simulink model "controller_arduino_4_mahdy_f"  (R2024a)
settings: Solver=FixedStepDiscrete  StartTime=0.0  StopTime=inf  FixedStep=0.01  RelTol=1e-3  EnableMultiTasking=on
libraries: arduinolib x15
settings Model: ExtModeTrigDuration=2  Creator=mahdy  LastModifiedBy=mahdy
settings SolverCC: AutoInsertRateTranBlk=on
settings OptimizationCC: EnhancedBackFolding=on  PassReuseOutputArgsAs=Individual arguments  ZeroExternalMemoryAtStartup=off  ZeroInternalMemoryAtStartup=off  MaxStackSize=64  OptimizeBlockOrder=speed  DifferentSizesBufferReuse=on  OptimizationCustomize=off  EfficientTunableParamExpr=on
settings DebuggingCC: ParameterTunabilityLossMsg=error
settings HardwareCC: ProdBitPerInt=16  ProdBitPerPointer=16  ProdBitPerSizeT=16  ProdBitPerPtrDiffT=16  ProdLargestAtomicFloat=None  ProdWordSize=8  ProdHWDeviceType=Atmel->AVR
settings SFSimCC: MATLABDynamicMemAlloc=off
settings RTWCC: Description=Embedded Coder  SystemTargetFile=ert.tlc  HardwareBoard=Arduino Uno  TemplateMakefile=ert_default_tmf  Toolchain=Arduino AVR  BuildConfiguration=Faster Runs
settings CodeAppCC: ForceParamTrailComments=on  IgnoreCustomStorageClasses=off  OperatorAnnotations=on  SimulinkDataObjDesc=on  SFDataObjDesc=on  InsertBlockDesc=on
settings ERTTargetCC: SupportContinuousTime=on  SupportVariableSizeSignals=on  ExtModeTransport=3  ExtModeStaticAlloc=on  ExtModeAutomaticAllocSize=off  ExtModeStaticAllocSize=250  ExtModeMexFile=ext_xcp  ExtModeIntrfLevel=Level2 - Open

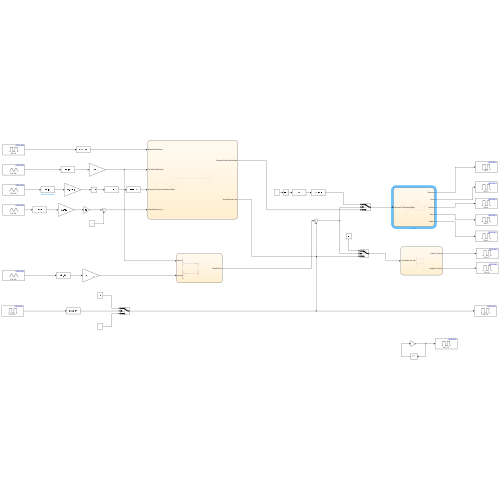
[thumbnail: Simulink's stored preview of the top-level diagram]
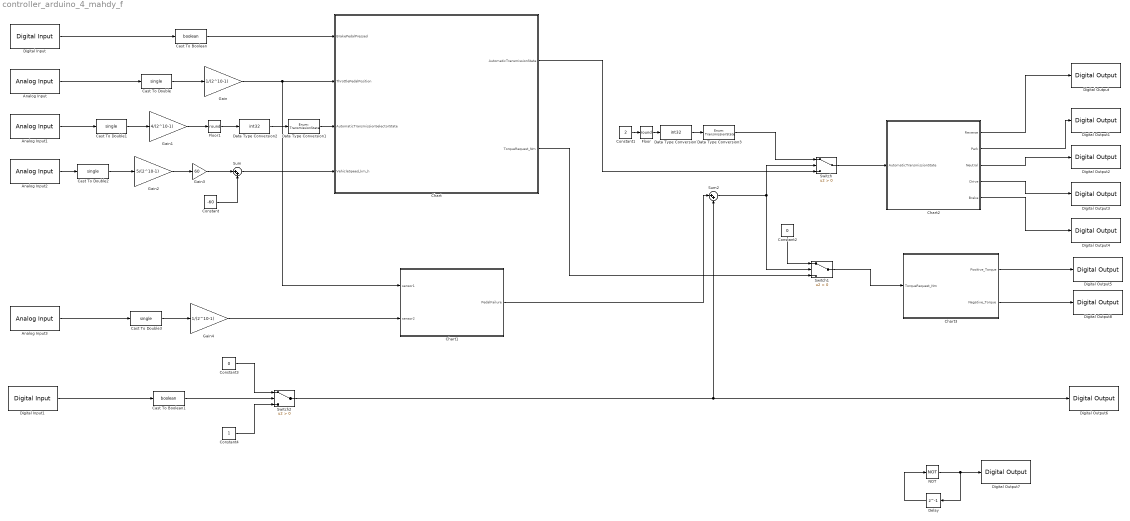
== system controller_arduino_4_mahdy_f ==
  Analog Input : arduinolib/Analog Input  pinNumber=2  ReadResultsOnly=off  ConversionTriggerSource=Software  ExternalTriggerType=uint32( 0 )  OutputDataType=uint16  EnableConversionCompleteNotify=off  EnableOuputStatus=off  SampleTime=-1  blockPlatform=arduino
  Analog Input1 : arduinolib/Analog Input  pinNumber=3  ReadResultsOnly=off  ConversionTriggerSource=Software  ExternalTriggerType=uint32( 0 )  OutputDataType=uint16  EnableConversionCompleteNotify=off  EnableOuputStatus=off  SampleTime=-1  blockPlatform=arduino
  Analog Input2 : arduinolib/Analog Input  pinNumber=4  ReadResultsOnly=off  ConversionTriggerSource=Software  ExternalTriggerType=uint32( 0 )  OutputDataType=uint16  EnableConversionCompleteNotify=off  EnableOuputStatus=off  SampleTime=-1  blockPlatform=arduino
  Analog Input3 : arduinolib/Analog Input  pinNumber=5  ReadResultsOnly=off  ConversionTriggerSource=Software  ExternalTriggerType=uint32( 0 )  OutputDataType=uint16  EnableConversionCompleteNotify=off  EnableOuputStatus=off  SampleTime=-1  blockPlatform=arduino
  Cast To Boolean : DataTypeConversion  OutDataTypeStr=boolean  SaturateOnIntegerOverflow=off  RndMeth=Floor
  Cast To Boolean1 : DataTypeConversion  OutDataTypeStr=boolean  SaturateOnIntegerOverflow=off  RndMeth=Floor
  Cast To Double{,1..3} (4 alike) : DataTypeConversion  OutDataTypeStr=single  SaturateOnIntegerOverflow=off  RndMeth=Floor
  Chart : Stateflow chart  TreatAsAtomicUnit=on
  Chart1 : Stateflow chart  TreatAsAtomicUnit=on
  Chart2 : Stateflow chart  TreatAsAtomicUnit=on
  Chart3 : Stateflow chart  TreatAsAtomicUnit=on
  Constant : Constant  Value=-60  OutDataTypeStr=single
  Constant1 : Constant  Value=2
  Constant2 : Constant  Value=0
  Constant3 : Constant  Value=0
  Constant4 : Constant
  Data Type Conversion1 : DataTypeConversion  OutDataTypeStr=Enum: TransmissionState  SaturateOnIntegerOverflow=off  RndMeth=Floor  LockScale=on
  Data Type Conversion2 : DataTypeConversion  OutDataTypeStr=int32  SaturateOnIntegerOverflow=off  RndMeth=Floor  LockScale=on
  Data Type Conversion3 : DataTypeConversion  OutDataTypeStr=Enum: TransmissionState  SaturateOnIntegerOverflow=off  RndMeth=Floor  LockScale=on
  Data Type Conversion7 : DataTypeConversion  OutDataTypeStr=int32  SaturateOnIntegerOverflow=off  RndMeth=Floor  LockScale=on
  Delay : Delay  DelayLength=1  SampleTime=0.01
  Digital Input : arduinolib/Digital Input  pinNumber=8  mode=Default  Direction=input  SampleTime=0.1  blockPlatform=arduino
  Digital Input1 : arduinolib/Digital Input  pinNumber=10  mode=Default  Direction=input  SampleTime=0.1  blockPlatform=arduino
  Digital Output : arduinolib/Digital Output  pinNumber=2  Direction=output  blockPlatform=arduino
  Digital Output1 : arduinolib/Digital Output  pinNumber=3  Direction=output  blockPlatform=arduino
  Digital Output2 : arduinolib/Digital Output  pinNumber=4  Direction=output  blockPlatform=arduino
  Digital Output3 : arduinolib/Digital Output  pinNumber=5  Direction=output  blockPlatform=arduino
  Digital Output4 : arduinolib/Digital Output  pinNumber=6  Direction=output  blockPlatform=arduino
  Digital Output5 : arduinolib/Digital Output  pinNumber=7  Direction=output  blockPlatform=arduino
  Digital Output6 : arduinolib/Digital Output  pinNumber=12  Direction=output  blockPlatform=arduino
  Digital Output7 : arduinolib/Digital Output  pinNumber=13  Direction=output  blockPlatform=arduino
  Digital Output8 : arduinolib/Digital Output  pinNumber=9  Direction=output  blockPlatform=arduino
  Floor : Rounding  Operator=round
  Floor1 : Rounding  Operator=round
  Gain : Gain  Gain=1/(2^10-1)
  Gain1 : Gain  Gain=4/(2^10-1)
  Gain2 : Gain  Gain=5/(2^10-1)
  Gain3 : Gain  Gain=60
  Gain4 : Gain  Gain=1/(2^10-1)
  NOT : Logic  Operator=NOT  IconShape=distinctive  AllPortsSameDT=off  OutDataTypeStr=boolean
  Sum : Sum  Inputs=|++
  Sum2 : Sum  Inputs=|++
  Switch : Switch  Criteria=u2 > Threshold  SaturateOnIntegerOverflow=off  InputSameDT=off
  Switch1 : Switch  Criteria=u2 > Threshold  SaturateOnIntegerOverflow=off  InputSameDT=off
  Switch2 : Switch  Criteria=u2 > Threshold  SaturateOnIntegerOverflow=off  InputSameDT=off
  wires:
  Digital Input/1 -> Cast To Boolean/1
  Cast To Boolean/1 -> Chart/1(BrakePedalPressed)
  Analog Input/1 -> Cast To Double/1
  Cast To Double/1 -> Gain/1
  Analog Input1/1 -> Cast To Double1/1
  Gain/1 -> Chart1/1(sensor1), Chart/2(ThrottlePedalPosition)
  Cast To Double1/1 -> Gain1/1
  Data Type Conversion2/1 -> Data Type Conversion1/1
  Floor1/1 -> Data Type Conversion2/1
  Data Type Conversion1/1 -> Chart/3(AutomaticTransmissionSelectorState)
  Gain1/1 -> Floor1/1
  Analog Input2/1 -> Cast To Double2/1
  Gain2/1 -> Gain3/1
  Cast To Double2/1 -> Gain2/1
  Gain3/1 -> Sum/1
  Constant/1 -> Sum/2
  Sum/1 -> Chart/4(VehicleSpeed_km_h)
  Analog Input3/1 -> Cast To Double3/1
  Cast To Double3/1 -> Gain4/1
  Gain4/1 -> Chart1/2(sensor2)
  Constant2/1 -> Switch1/1
  Data Type Conversion3/1 -> Switch/1
  Sum2/1 -> Switch/2, Switch1/2
  Data Type Conversion7/1 -> Data Type Conversion3/1
  Chart1/1(PedalFailure) -> Sum2/1
  Chart/2(TorqueRequest_Nm) -> Switch1/3
  Chart/1(AutomaticTransmissionState) -> Switch/3
  NOT/1 -> Delay/1, Digital Output7/1
  Delay/1 -> NOT/1
  Digital Input1/1 -> Cast To Boolean1/1
  Constant3/1 -> Switch2/1
  Constant4/1 -> Switch2/3
  Switch2/1 -> Digital Output6/1, Sum2/2
  Chart3/2(Negative_Torque) -> Digital Output8/1
  Chart3/1(Positive_Torque) -> Digital Output5/1
  Switch1/1 -> Chart3/1(TorqueRequest_Nm)
  Switch/1 -> Chart2/1(AutomaticTransmissionState)
  Chart2/2(Park) -> Digital Output1/1
  Chart2/3(Neutral) -> Digital Output2/1
  Chart2/1(Reverse) -> Digital Output/1
  Chart2/5(Brake) -> Digital Output4/1
  Constant1/1 -> Floor/1
  Floor/1 -> Data Type Conversion7/1
  Chart2/4(Drive) -> Digital Output3/1
  Cast To Boolean1/1 -> Switch2/2

== stateflow chart controller_arduino_4_mahdy_f/Chart2 ==
  settings: updateMethod=DISCRETE  sampleTime=0.1
  state ReverseState
    entry:
    Reverse = 1
  state BrakeState
    entry:
    Brake = 1
  state ParkState
    entry:
    Park = 1
  state Input_transmissionState
  state NeutralState
    entry:
    Neutral = 1
  state DriveState
    entry:
    Drive = 1
  ReverseState -> Input_transmissionState : [AutomaticTransmissionState ~= TransmissionState.Reverse]{Reverse = 0}
  Input_transmissionState -> ReverseState [order 1] : [AutomaticTransmissionState == TransmissionState.Reverse]
  (default) -> Input_transmissionState
  Input_transmissionState -> BrakeState [order 5] : [AutomaticTransmissionState == TransmissionState.Brake]
  BrakeState -> Input_transmissionState : [AutomaticTransmissionState ~= TransmissionState.Brake]{Brake = 0}
  Input_transmissionState -> ParkState [order 2] : [AutomaticTransmissionState == TransmissionState.Park]
  ParkState -> Input_transmissionState : [AutomaticTransmissionState ~= TransmissionState.Park]{Park = 0}
  Input_transmissionState -> DriveState [order 4] : [AutomaticTransmissionState == TransmissionState.Drive]
  DriveState -> Input_transmissionState : [AutomaticTransmissionState ~= TransmissionState.Drive]{Drive = 0}
  Input_transmissionState -> NeutralState [order 3] : [AutomaticTransmissionState == TransmissionState.Neutral]
  NeutralState -> Input_transmissionState : [AutomaticTransmissionState ~= TransmissionState.Neutral]{Neutral = 0}
  data: AutomaticTransmissionState input; Reverse output =0; Park output =0; Neutral output =0; Drive output =0; Brake output =0

== stateflow chart controller_arduino_4_mahdy_f/Chart ==
  settings: updateMethod=DISCRETE  sampleTime=0.1
  state Reverse
    entry:
    AutomaticTransmissionState =TransmissionState. Reverse;
    during:
    TorqueRequest_Nm = -ThrottlePedalPosition*MAX_TORQUE_REVERSE;
  state Park
    entry:
    AutomaticTransmissionState = TransmissionState.Park;
    TorqueRequest_Nm = 0;
  state Neutral
    entry:
    AutomaticTransmissionState = TransmissionState.Neutral;
    TorqueRequest_Nm = 0;
  state Bmode
    entry:
    AutomaticTransmissionState = TransmissionState.Brake;
    state Acceleration
      during:
      TorqueRequest_Nm =MAX_TORQUE*(ThrottlePedalPosition-1/3)*3/2;
    state Regenerative_Braking
      during:
      TorqueRequest_Nm =- MAX_TORQUE*(1-3*ThrottlePedalPosition)
    state Stop
      entry:
      TorqueRequest_Nm = 0;
    (default) -> Acceleration
    Acceleration -> Regenerative_Braking : [ThrottlePedalPosition<=1/3]
    Regenerative_Braking -> Acceleration [order 1] : [ThrottlePedalPosition>1/3]
    Stop -> Acceleration : [ThrottlePedalPosition>1/3]
    Regenerative_Braking -> Stop [order 2] : [ 0<ThrottlePedalPosition<=1/3 &&VehicleSpeed_km_h<=0.05 ]
  state Drive
    entry:
    AutomaticTransmissionState = TransmissionState.Drive;
    during:
    TorqueRequest_Nm = ThrottlePedalPosition*MAX_TORQUE;
  Reverse -> Neutral : [AutomaticTransmissionSelectorState ==TransmissionState. Neutral || AutomaticTransmissionSelectorState ==TransmissionState. Drive ||AutomaticTransmissionSelectorState ==TransmissionState. Brake||AutomaticTransmissionSelectorState ==TransmissionState. Park]
  Neutral -> Reverse [order 3] : [ VehicleSpeed_km_h<5 && AutomaticTransmissionSelectorState ==TransmissionState. Reverse &&BrakePedalPressed ==1]
  (default) -> Park
  Neutral -> Park [order 2] : [BrakePedalPressed ==1 && abs(VehicleSpeed_km_h)<5 && AutomaticTransmissionSelectorState == TransmissionState.Park]
  Park -> Neutral : [BrakePedalPressed ==1 && (AutomaticTransmissionSelectorState == TransmissionState.Reverse||AutomaticTransmissionSelectorState == TransmissionState.Neutral || AutomaticTransmissionSelectorState==TransmissionState.Brake|| AutomaticTransmissionSelectorState == TransmissionState.Drive)]
  Drive -> Neutral [order 1] : [AutomaticTransmissionSelectorState ==TransmissionState. Neutral||AutomaticTransmissionSelectorState == TransmissionState.Reverse||AutomaticTransmissionSelectorState == TransmissionState.Park]
  Neutral -> Drive [order 1] : [BrakePedalPressed==1 && VehicleSpeed_km_h>-5 && AutomaticTransmissionSelectorState ==TransmissionState. Drive || AutomaticTransmissionSelectorState == TransmissionState.Brake ]
  Drive -> Bmode [order 2] : [AutomaticTransmissionSelectorState == TransmissionState.Brake ]
  Bmode -> Drive : [AutomaticTransmissionSelectorState == TransmissionState.Drive||AutomaticTransmissionSelectorState == TransmissionState.Neutral||AutomaticTransmissionSelectorState == TransmissionState.Reverse||AutomaticTransmissionSelectorState == TransmissionState.Park]
  data: BrakePedalPressed input boolean; ThrottlePedalPosition input single; AutomaticTransmissionSelectorState input Enum: TransmissionState; VehicleSpeed_km_h input single; AutomaticTransmissionState output Enum: TransmissionState; TorqueRequest_Nm output single; MAX_TORQUE_REVERSE local =40; MAX_TORQUE local =80

== stateflow chart controller_arduino_4_mahdy_f/Chart3 ==
  (default) -> (junction 7) : % Torque_request
  (junction 7) -> (junction 8) [order 1] : [TorqueRequest_Nm>=0]
  (junction 7) -> (junction 9) [order 2] : {Positive_Torque=0;Negative_Torque=1}
  (junction 8) -> (junction 10) : {Positive_Torque = 1;Negative_Torque = 0}
  (junction 10) -> (junction 9)
  (junction 9) -> (junction 11)
  data: TorqueRequest_Nm input; Positive_Torque output; Negative_Torque output

== stateflow chart controller_arduino_4_mahdy_f/Chart1 ==
  settings: updateMethod=DISCRETE  sampleTime=0.1
  (default) -> (junction 22) : % PedalSensorFailure
  (junction 22) -> (junction 23) [order 1] : [sensor1-sensor2>=0.05|| error == 1]
  (junction 22) -> (junction 24) [order 2] : {PedalFailure=0;error = 0}
  (junction 23) -> (junction 25) : {PedalFailure=1;error=1}
  (junction 25) -> (junction 24)
  (junction 24) -> (junction 26)
  data: sensor1 input; sensor2 input; PedalFailure output; error local =0
